simulink model "hw1_2"  (R2018a)
settings: Solver=VariableStepAuto  StartTime=0.0  StopTime=50  RelTol=1e-3
settings Model: Creator=Halil Temurtaş  LastModifiedBy=Halil Temurtaş

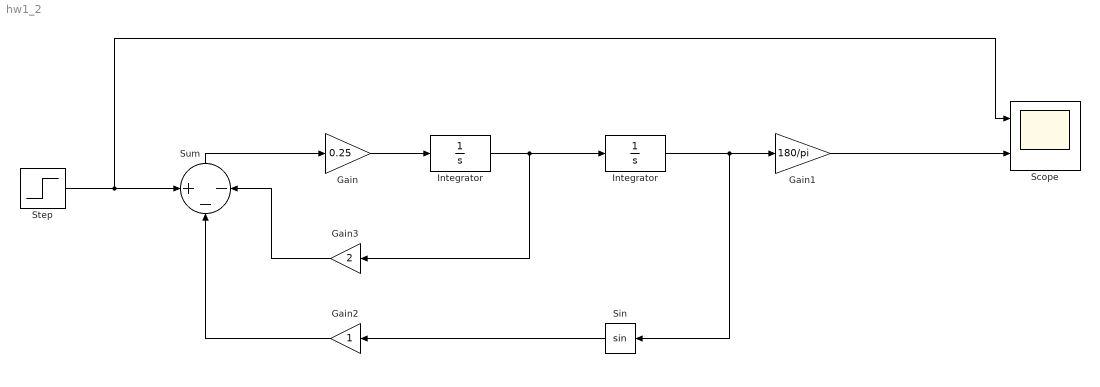
== system hw1_2 ==
  Gain : Gain  Gain=0.25
  Gain1 : Gain  Gain=180/pi
  Gain2 : Gain
  Gain3 : Gain  Gain=2
  Integrator : TransferFcn  Denominator=[1 0]
  "Integrator " : TransferFcn  Denominator=[1 0]
  Scope : Scope  NumInputPorts=2
  Sin : Trigonometry
  Step : Step  Time=0  After=15  SampleTime=0
  Sum : Sum  Inputs=+--
  wires:
  Step/1 -> Scope/1, Sum/1
  Sum/1 -> Gain/1
  Gain3/1 -> Sum/3
  Gain2/1 -> Sum/2
  Gain/1 -> Integrator/1
  Integrator/1 -> Gain3/1, "Integrator "/1
  "Integrator "/1 -> Sin/1, Gain1/1
  Gain1/1 -> Scope/2
  Sin/1 -> Gain2/1
